simulink model "ControlSystem"  (R2023a)
settings: Solver=VariableStepAuto  StartTime=0.0  StopTime=4  RelTol=1e-3
values from neighbouring files (symbols this model uses):
  ak0 = 1    [main.m]
  ak1 = 0.5    [main.m]
  ap0 = 1    [main.m]
  ap1 = 0.001    [main.m]
  bk0 = 0    [main.m]
  bk1 = 0.5    [main.m]
  bp0 = 1    [main.m]
  bp1 = 0.001    [main.m]
  Kc = 0.0015    [main.m]
  Ki = 0.0003    [main.m]
  kip = 0    [main.m]
  Kk = 22500    [main.m]
  kpd = 0    [main.m]
  kpid = 1    [main.m]
settings Model: Creator=ycheb  LastModifiedBy=ycheb

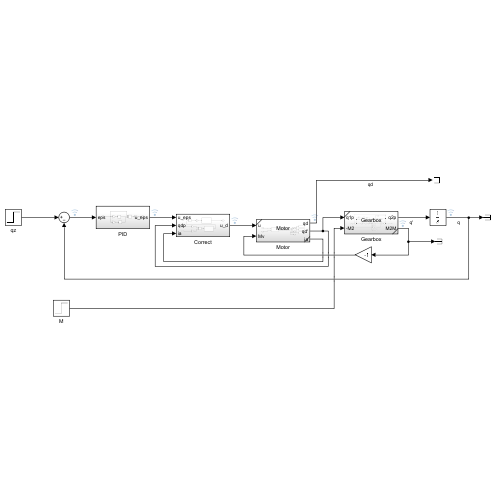
[thumbnail: Simulink's stored preview of the top-level diagram]
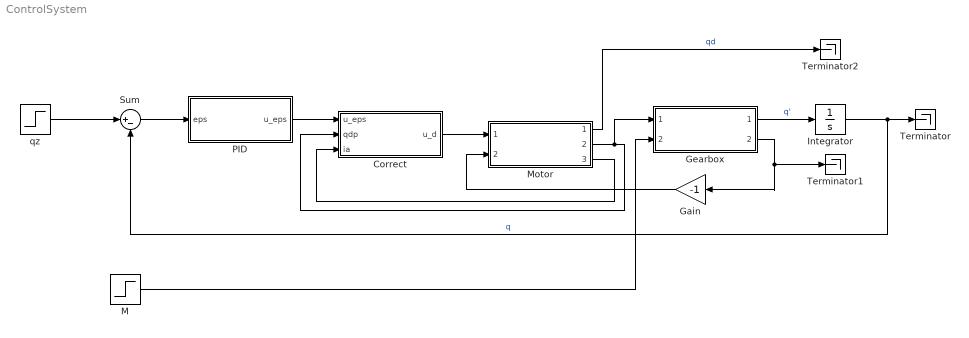
== system ControlSystem ==
  Correct : Subsystem
  Gain : Gain  Gain=-1
  Gearbox : Subsystem  ReferencedSubsystem=Gearbox
  Integrator : Integrator
  M : Step  Time=0  After=0  SampleTime=0
  Motor : Subsystem  ReferencedSubsystem=Motor
  PID : Subsystem
  Sum : Sum  Inputs=|+-
  Terminator : Terminator
  Terminator1 : Terminator
  Terminator2 : Terminator
  qz : Step  Time=0  After=0.1  SampleTime=0
  wires:
  Gearbox/1 -> Integrator/1  "q'"
  Correct/1(u_d) -> Motor/1
  PID/1(u_eps) -> Correct/1(u_eps)
  Motor/3 -> Correct/3(ia)
  Motor/2 -> Gearbox/1, Correct/2(qdp)
  M/1 -> Gearbox/2
  Gearbox/2 -> Terminator1/1, Gain/1
  Integrator/1 -> Sum/2, Terminator/1  "q"
  qz/1 -> Sum/1
  Sum/1 -> PID/1(eps)
  Motor/1 -> Terminator2/1  "qd"
  Gain/1 -> Motor/2

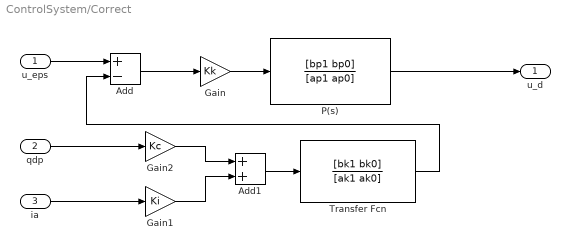
== system ControlSystem/Correct ==
  u_eps : Inport
  qdp : Inport  Port=2
  ia : Inport  Port=3
  Add : Sum  Inputs=+-
  Add1 : Sum
  Gain : Gain  Gain=Kk
  Gain1 : Gain  Gain=Ki
  Gain2 : Gain  Gain=Kc
  P(s) : TransferFcn  Numerator=[bp1 bp0]  Denominator=[ap1 ap0]
  Transfer Fcn : TransferFcn  Numerator=[bk1 bk0]  Denominator=[ak1 ak0]
  u_d : Outport
  wires:
  u_eps/1 -> Add/1
  Add/1 -> Gain/1
  Gain/1 -> P(s)/1
  P(s)/1 -> u_d/1
  ia/1 -> Gain1/1
  qdp/1 -> Gain2/1
  Gain2/1 -> Add1/1
  Gain1/1 -> Add1/2
  Add1/1 -> Transfer Fcn/1
  Transfer Fcn/1 -> Add/2

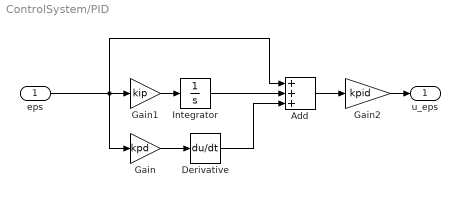
== system ControlSystem/PID ==
  eps : Inport
  Add : Sum  Inputs=+++
  Derivative : Derivative
  Gain : Gain  Gain=kpd
  Gain1 : Gain  Gain=kip
  Gain2 : Gain  Gain=kpid
  Integrator : Integrator
  u_eps : Outport
  wires:
  Gain/1 -> Derivative/1
  Integrator/1 -> Add/2
  Derivative/1 -> Add/3
  eps/1 -> Gain/1, Add/1, Gain1/1
  Gain1/1 -> Integrator/1
  Add/1 -> Gain2/1
  Gain2/1 -> u_eps/1
